simulink model "motor_model_7__az"  (R2018b)
settings: Solver=VariableStepAuto  StartTime=0.0  StopTime=1  RelTol=1e-3
model workspace (MAT data in the model file):
  A1 = 0.209333333333
  A2 = 0.0330526315789
  K = 700
  Km = 3.29
  Kn = 3.7
  Mn = 2.14
  T1 = 0.05
  T2 = 5e-05
  Te = 0.0001
  Tm = 1.08
  Tpwm = 6.25e-05
  U = 27
  dangle = 0.000383
  dt = 0.5
  dx = 3.14
  max = 3.14
  min = -3.14
  omega1 = 1.005
  omega2 = 6.28
  target = 3.14
  w = 0.209333333333
libraries: simulink x2
settings Model: Creator=Sainquake  LastModifiedBy=Sainquake

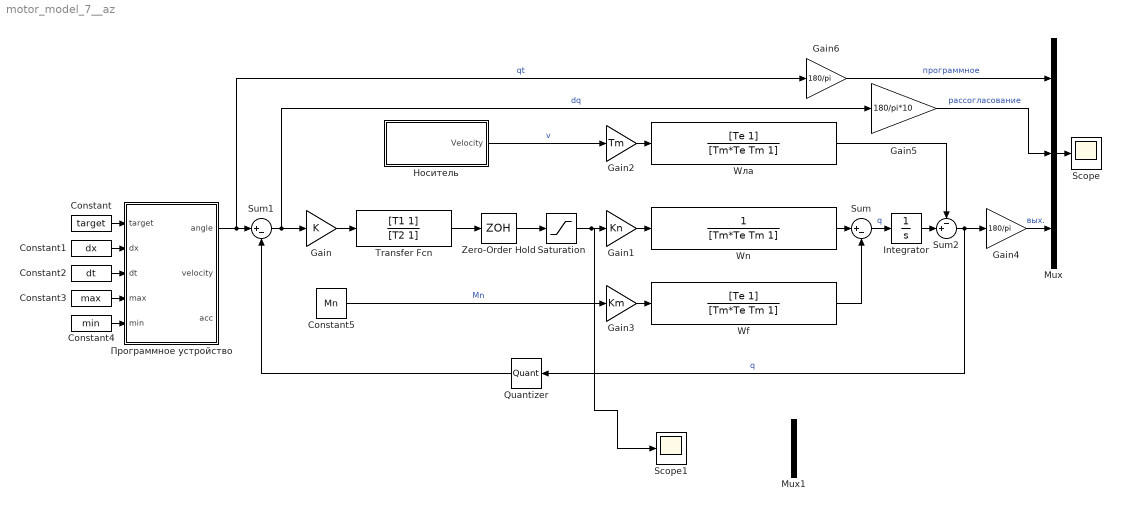
== system motor_model_7__az ==
  Constant : Constant  Value=target
  Constant1 : Constant  Value=dx
  Constant2 : Constant  Value=dt
  Constant3 : Constant  Value=max
  Constant4 : Constant  Value=min
  Constant5 : Constant  Value=Mn
  Gain : Gain  Gain=K
  Gain1 : Gain  Gain=Kn
  Gain2 : Gain  Gain=Tm
  Gain3 : Gain  Gain=Km
  Gain4 : Gain  Gain=180/pi
  Gain5 : Gain  Gain=180/pi*10
  Gain6 : Gain  Gain=180/pi
  Integrator : Integrator
  Mux : Mux  Inputs=3
  Mux1 : Mux  Inputs=3
  Quantizer : Quantizer  QuantizationInterval=dangle*4
  Saturation : Saturate  UpperLimit=U/2  LowerLimit=-U/2
  Scope : Scope
  Scope1 : Scope
  Sum : Sum  Inputs=|+-
  Sum1 : Sum  Inputs=|+-
  Sum2 : Sum  Inputs=-+|
  Transfer Fcn : TransferFcn  Numerator=[T1 1]  Denominator=[T2 1]
  Wf : TransferFcn  Numerator=[Te 1]  Denominator=[Tm*Te Tm 1]
  "Wn " : TransferFcn  Denominator=[Tm*Te Tm 1]
  Wла : TransferFcn  Numerator=[Te 1]  Denominator=[Tm*Te Tm 1]
  Zero-Order Hold : ZeroOrderHold  SampleTime=Tpwm
  Носитель : Subsystem
  Программное устройство : Subsystem
  wires:
  Sum/1 -> Integrator/1  "q"
  Sum1/1 -> Gain5/1, Gain/1  "dq"
  Программное устройство/1(angle) -> Gain6/1, Sum1/1  "qt"
  Sum2/1 -> Quantizer/1, Gain4/1  "q"
  Constant5/1 -> Gain3/1  "Mn"
  Носитель/1(Velocity) -> Gain2/1  "v"
  Constant/1 -> Программное устройство/1(target)
  Constant1/1 -> Программное устройство/2("dx ")
  Constant2/1 -> Программное устройство/3(dt)
  Constant4/1 -> Программное устройство/5(min)
  Constant3/1 -> Программное устройство/4(max)
  Gain/1 -> Transfer Fcn/1
  Integrator/1 -> Sum2/2
  "Wn "/1 -> Sum/1
  Wла/1 -> Sum2/1
  Wf/1 -> Sum/2
  Gain1/1 -> "Wn "/1
  Gain2/1 -> Wла/1
  Gain3/1 -> Wf/1
  Gain4/1 -> Mux/3  "вых."
  Gain5/1 -> Mux/2  "рассогласование"
  Gain6/1 -> Mux/1  "программное"
  Mux/1 -> Scope/1
  Transfer Fcn/1 -> Zero-Order Hold/1
  Quantizer/1 -> Sum1/2
  Saturation/1 -> Scope1/1, Gain1/1
  Zero-Order Hold/1 -> Saturation/1

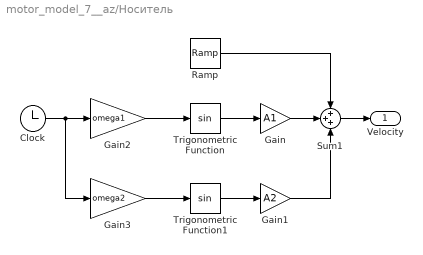
== system motor_model_7__az/Носитель ==
  Clock : Clock
  Gain : Gain  Gain=A1
  Gain1 : Gain  Gain=A2
  Gain2 : Gain  Gain=omega1
  Gain3 : Gain  Gain=omega2
  Ramp : simulink/Sources/Ramp  slope=w  start=0  InitialOutput=0
  Sum1 : Sum  Inputs=+++
  Trigonometric Function : Trigonometry
  Trigonometric Function1 : Trigonometry
  Velocity : Outport
  wires:
  Trigonometric Function/1 -> Gain/1
  Trigonometric Function1/1 -> Gain1/1
  Clock/1 -> Gain2/1, Gain3/1
  Gain2/1 -> Trigonometric Function/1
  Gain3/1 -> Trigonometric Function1/1
  Gain/1 -> Sum1/2
  Gain1/1 -> Sum1/3
  Sum1/1 -> Velocity/1
  Ramp/1 -> Sum1/1

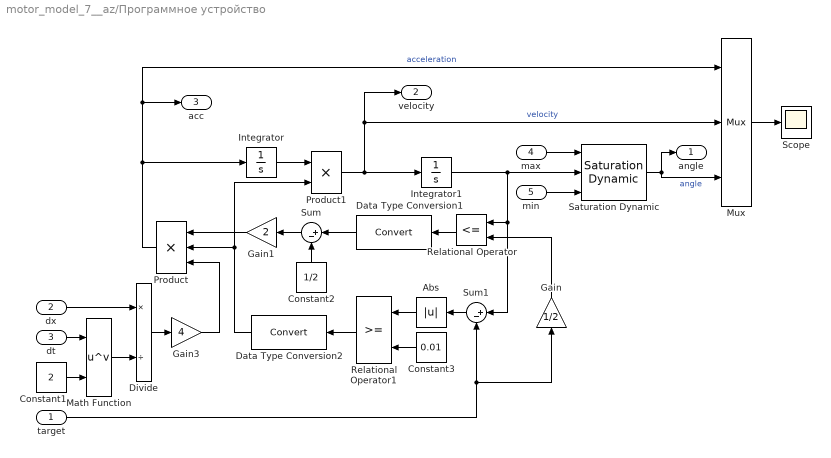
== system motor_model_7__az/Программное устройство ==
  target : Inport
  "dx " : Inport  Port=2
  dt : Inport  Port=3
  max : Inport  Port=4
  min : Inport  Port=5
  Abs : Abs
  Constant1 : Constant  Value=2
  Constant2 : Constant  Value=1/2
  Constant3 : Constant  Value=0.01
  Data Type Conversion1 : DataTypeConversion
  Data Type Conversion2 : DataTypeConversion
  Divide : Product  Inputs=*/
  Gain : Gain  Gain=1/2
  Gain1 : Gain  Gain=2
  Gain3 : Gain  Gain=4
  Integrator : Integrator
  Integrator1 : Integrator
  Math Function : Math  Operator=pow  SaturateOnIntegerOverflow=on
  Mux : Mux  Inputs=3
  Product : Product  Inputs=3
  Product1 : Product
  Relational Operator : RelationalOperator  Operator=<=  OutDataTypeStr=boolean  RndMeth=Simplest
  Relational Operator1 : RelationalOperator  OutDataTypeStr=boolean  RndMeth=Simplest
  Saturation Dynamic : simulink/Discontinuities/Saturation Dynamic  OutMin=[]  OutMax=[]  OutDataTypeStr=Inherit: Same as second input  OutDataType=fixdt(1, 16)  OutScaling=2^-10  DoSatur=off
  Scope : Scope
  Sum : Sum  Inputs=|+-
  Sum1 : Sum  Inputs=|+-
  angle : Outport
  velocity : Outport  Port=2
  acc : Outport  Port=3
  wires:
  "dx "/1 -> Divide/1
  Constant1/1 -> Math Function/2
  Gain3/1 -> Product/3
  Data Type Conversion1/1 -> Sum/1
  Sum/1 -> Gain1/1
  Product/1 -> Integrator/1, Mux/1, acc/1  "acceleration"
  Product1/1 -> Integrator1/1, Mux/2, velocity/1  "velocity"
  Abs/1 -> Relational Operator1/1
  Relational Operator1/1 -> Data Type Conversion2/1
  Sum1/1 -> Abs/1
  Data Type Conversion2/1 -> Product1/2, Product/2
  Divide/1 -> Gain3/1
  Constant2/1 -> Sum/2
  Integrator/1 -> Product1/1
  target/1 -> Gain/1, Sum1/2
  Math Function/1 -> Divide/2
  Gain/1 -> Relational Operator/2
  Integrator1/1 -> Sum1/1, Relational Operator/1, Saturation Dynamic/2
  Mux/1 -> Scope/1
  Gain1/1 -> Product/1
  Relational Operator/1 -> Data Type Conversion1/1
  dt/1 -> Math Function/1
  Constant3/1 -> Relational Operator1/2
  max/1 -> Saturation Dynamic/1
  min/1 -> Saturation Dynamic/3
  Saturation Dynamic/1 -> Mux/3, angle/1  "angle"
